simulink model "lab7"  (R2016a)
settings: Solver=ode45  StartTime=0.0  StopTime=15  MaxStep=0.02  MinStep=0.01  RelTol=1e-3
libraries: simulink x1
settings Model: Creator=ms36124  LastModifiedBy=ms36124
settings SolverCC: InitialStep=0.01

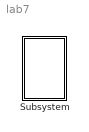
== system lab7 ==
  Subsystem : Subsystem  mask{n=3, g=9.81, k=1, m=2, l=4, x=-1, y=-1, xi=[-1 1 1], yi=[1 1 -1], di=[0.1 0.1 0.1], ai=[1 -1 1.5]}

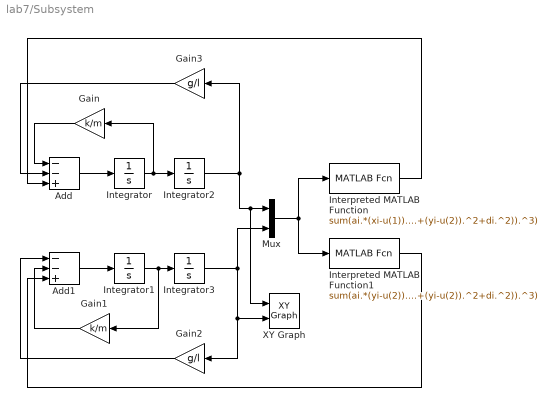
== system lab7/Subsystem ==
  Add : Sum  Inputs=--+
  Add1 : Sum  Inputs=--+
  Gain : Gain  Gain=k/m
  Gain1 : Gain  Gain=k/m
  Gain2 : Gain  Gain=g/l
  Gain3 : Gain  Gain=g/l
  Integrator : Integrator
  Integrator1 : Integrator
  Integrator2 : Integrator  InitialCondition=x
  Integrator3 : Integrator  InitialCondition=y
  Interpreted MATLAB Function : MATLABFcn  MATLABFcn=sum(ai.*(xi-u(1))./(sqrt((xi-u(1)).^2+(yi-u(2)).^2+di.^2)).^3)  OutputDimensions=1
  Interpreted MATLAB Function1 : MATLABFcn  MATLABFcn=sum(ai.*(yi-u(2))./(sqrt((xi-u(1)).^2+(yi-u(2)).^2+di.^2)).^3)  OutputDimensions=1
  Mux : Mux  Inputs=2
  XY Graph : simulink/Sinks/XY Graph  xmin=-1  xmax=1  ymin=-1  ymax=1  st=-1
  wires:
  Integrator2/1 -> XY Graph/1, Mux/1, Gain3/1
  Integrator3/1 -> XY Graph/2, Gain2/1, Mux/2
  Gain3/1 -> Add/2
  Gain2/1 -> Add1/1
  Gain1/1 -> Add1/2
  Interpreted MATLAB Function/1 -> Add/3
  Gain/1 -> Add/1
  Interpreted MATLAB Function1/1 -> Add1/3
  Mux/1 -> Interpreted MATLAB Function1/1, Interpreted MATLAB Function/1
  Add/1 -> Integrator/1
  Add1/1 -> Integrator1/1
  Integrator/1 -> Gain/1, Integrator2/1
  Integrator1/1 -> Gain1/1, Integrator3/1
